simulink model "MySimModel"  (R2024b)
settings: Solver=VariableStepAuto  StartTime=0.0  StopTime=10.0  RelTol=1e-3
undefined symbols (not defined in the file): DiscIntNeverNeededParam
settings Model: Creator=xinxing  LastModifiedBy=xinxing

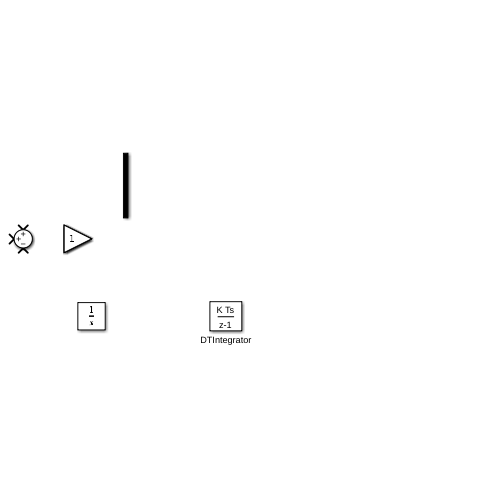
[thumbnail: Simulink's stored preview of the top-level diagram]
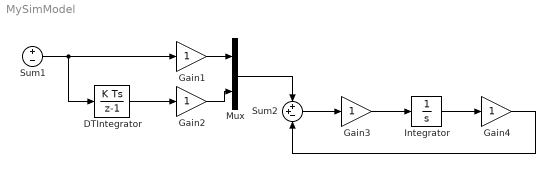
== system MySimModel ==
  DTIntegrator : DiscreteIntegrator  SampleTime=-1  ICPrevOutput=DiscIntNeverNeededParam  ICPrevScaledInput=DiscIntNeverNeededParam
  Gain{1..4} (4 alike) : Gain
  Integrator : Integrator
  Mux : Mux  Inputs=2
  Sum1 : Sum  Inputs=+-
  Sum2 : Sum  Inputs=++-
  wires:
  Gain4/1 -> Sum2/3
  Sum2/1 -> Gain3/1
  Mux/1 -> Sum2/1
  Gain2/1 -> Mux/2
  Integrator/1 -> Gain4/1
  Gain1/1 -> Mux/1
  DTIntegrator/1 -> Gain2/1
  Gain3/1 -> Integrator/1
  Sum1/1 -> DTIntegrator/1, Gain1/1
